simulink model "donghocnguoc_vantoc"  (R2023b)
settings: Solver=FixedStepAuto  StartTime=0.0  StopTime=7  FixedStep=0.01  RelTol=1e-3
settings Model: Creator=DELL  LastModifiedBy=DELL

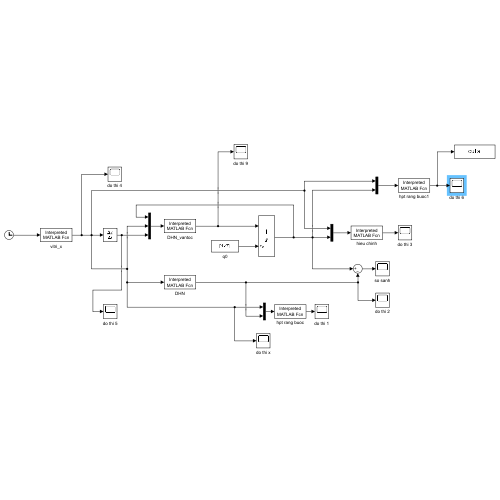
[thumbnail: Simulink's stored preview of the top-level diagram]
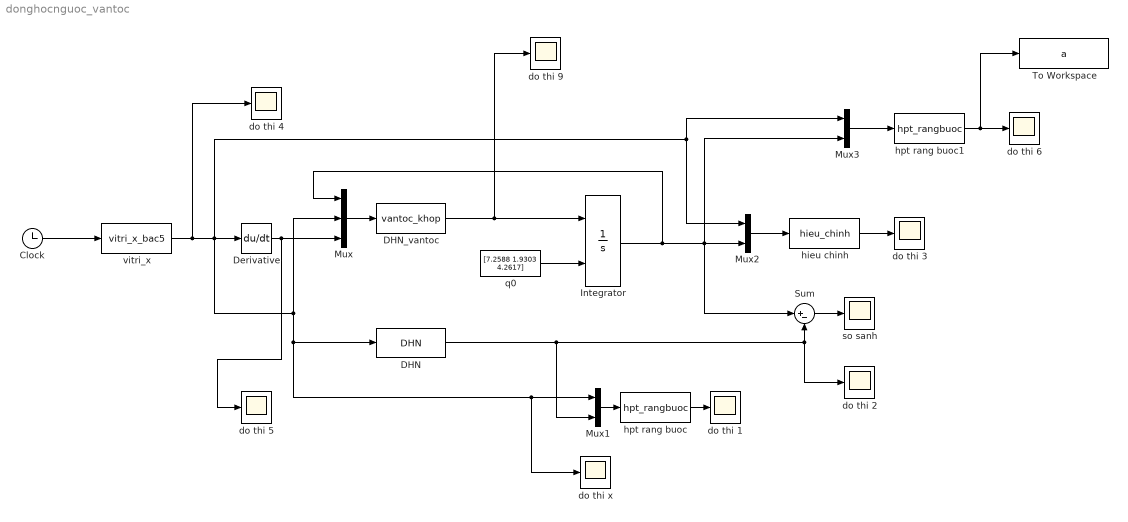
== system donghocnguoc_vantoc ==
  Clock : Clock
      settings: Decimation=2
  DHN : MATLABFcn  MATLABFcn=DHN  OutputDimensions=3  OutputSignalType=real  Output1D=off
  DHN_vantoc : MATLABFcn  MATLABFcn=vantoc_khop  OutputDimensions=3  OutputSignalType=real  Output1D=off
  Derivative : Derivative
  Integrator : Integrator  InitialConditionSource=external
  Mux : Mux  Inputs=3
  Mux1 : Mux  Inputs=2
  Mux2 : Mux  Inputs=2
  Mux3 : Mux  Inputs=2
  Sum : Sum  Inputs=|+-
  To Workspace : ToWorkspace  VariableName=a  SaveFormat=Timeseries  SampleTime=-1
  do thi {1..6,9} (7 alike) : Scope
  do thi x : Scope
  hieu chinh : MATLABFcn  MATLABFcn=hieu_chinh
  hpt rang buoc : MATLABFcn  MATLABFcn=hpt_rangbuoc
  hpt rang buoc1 : MATLABFcn  MATLABFcn=hpt_rangbuoc
  q0 : Constant  Value="[7.2588    1.9303    4.2617]"
  so sanh : Scope
  vitri_x : MATLABFcn  MATLABFcn=vitri_x_bac5  OutputDimensions=3
  wires:
  DHN_vantoc/1 -> do thi 9/1, Integrator/1
  Integrator/1 -> Mux/1, Mux2/2, Mux3/2, Sum/1
  Mux/1 -> DHN_vantoc/1
  q0/1 -> Integrator/2
  vitri_x/1 -> do thi 4/1, Mux2/1, Mux3/1, do thi x/1, Mux1/1, DHN/1, Mux/2, Derivative/1
  DHN/1 -> Mux1/2, do thi 2/1, Sum/2
  Derivative/1 -> do thi 5/1, Mux/3
  Sum/1 -> so sanh/1
  Mux2/1 -> hieu chinh/1
  Mux1/1 -> hpt rang buoc/1
  hpt rang buoc/1 -> do thi 1/1
  hieu chinh/1 -> do thi 3/1
  Clock/1 -> vitri_x/1
  Mux3/1 -> hpt rang buoc1/1
  hpt rang buoc1/1 -> To Workspace/1, do thi 6/1
